simulink model "II"  (Simulink 8.8)
settings: Solver=VariableStepAuto  StartTime=0.0  StopTime=10.0  RelTol=1e-3
libraries: dsparch4 x1
settings Model: SuppressorTable=22 serialization::archive 11 0 6 0 0 0 8 0  Creator=User  LastModifiedBy=User
settings DataIOCC: LimitDataPoints=off  SaveFormat=Dataset  SignalLoggingSaveFormat=Dataset
settings OptimizationCC: LifeSpan=auto
settings DebuggingCC: UnderspecifiedInitializationDetection=Simplified  MergeDetectMultiDrivingBlocksExec=error  FcnCallInpInsideContextMsg=error  StateNameClashWarn=none  SFUnexpectedBacktrackingDiag=error  SFNoUnconditionalDefaultTransitionDiag=error  SFExecutionAtInitializationDiag=warning
settings HardwareCC: ProdBitPerPointer=64  ProdBitPerSizeT=64  ProdBitPerPtrDiffT=64  ProdLargestAtomicFloat=Float  ProdIntDivRoundTo=Zero  ProdEndianess=LittleEndian  ProdWordSize=64  ProdHWDeviceType=Intel->x86-64 (Windows64)
settings ModelReferenceCC: PropagateSignalLabelsOutOfModel=on
settings GRTTargetCC: TargetLangStandard=C99 (ISO)  GeneratePreprocessorConditionals=Use local settings  CombineOutputUpdateFcns=on  GRTInterface=off
settings ConfigComp: CovMetricSettings=dwe  CovHtmlReporting=off  CovSaveCumulativeToWorkspaceVar=off  CovSaveSingleToWorkspaceVar=off  CovExternalEMLEnable=on

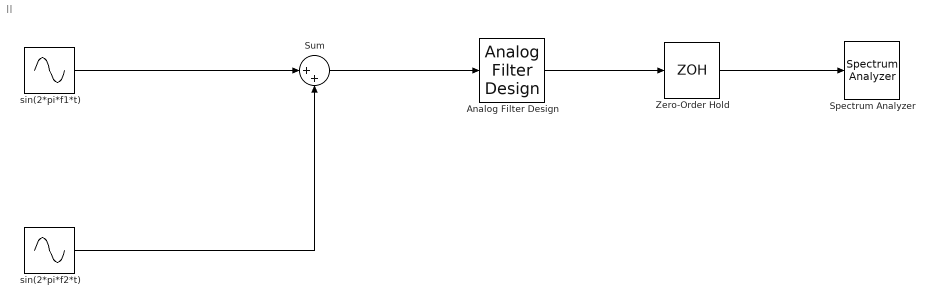
== system II ==
  Analog Filter Design : dsparch4/Analog Filter Design  method=Butterworth  filttype=Lowpass  N=8  Wlo=2*pi*200  Whi=80  Rp=2  Rs=40
  Spectrum Analyzer : SpectrumAnalyzer
  Sum : Sum  Inputs=|++
  Zero-Order Hold : ZeroOrderHold  SampleTime=0.0025
  sin(2*pi*f1*t) : Sin  Frequency=2*pi*100  SampleTime=0
  sin(2*pi*f2*t) : Sin  Frequency=2*pi*160  SampleTime=0
  wires:
  sin(2*pi*f1*t)/1 -> Sum/1
  sin(2*pi*f2*t)/1 -> Sum/2
  Sum/1 -> Analog Filter Design/1
  Analog Filter Design/1 -> Zero-Order Hold/1
  Zero-Order Hold/1 -> Spectrum Analyzer/1
